simulink model "untitledtoch"  (R2016b)
settings: Solver=VariableStepAuto  StartTime=0  StopTime=20  MaxStep=0.001  RelTol=1e-3
libraries: simulink x1
settings Model: Creator=Admin  LastModifiedBy=Admin

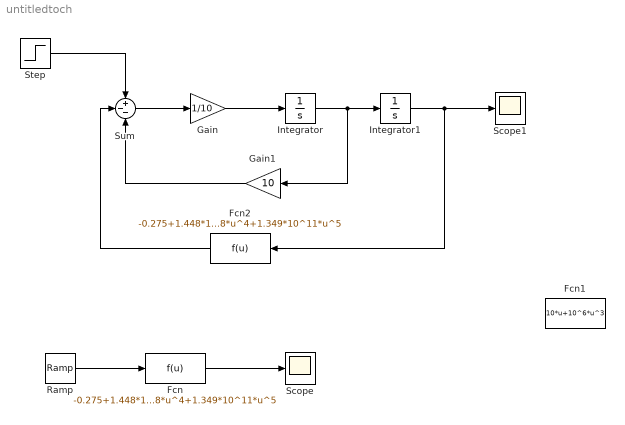
== system untitledtoch ==
  Fcn : Fcn  Expr=-0.275+1.448*10^3*u+-4.325*10^4*u^2+-1.543*10^7*u^3+2.141*10^8*u^4+1.349*10^11*u^5
  Fcn1 : Fcn  Expr=10*u+10^6*u^3
  Fcn2 : Fcn  Expr=-0.275+1.448*10^3*u+-4.325*10^4*u^2+-1.543*10^7*u^3+2.141*10^8*u^4+1.349*10^11*u^5
  Gain : Gain  Gain=1/10
  Gain1 : Gain  Gain=10
  Integrator : Integrator
  Integrator1 : Integrator
  Ramp : simulink/Sources/Ramp  slope=0.012  start=0  X0=-0.01
  Scope : Scope
  Scope1 : Scope
  Step : Step  Time=0  SampleTime=0
  Sum : Sum  Inputs=+--
  wires:
  Ramp/1 -> Fcn/1
  Fcn/1 -> Scope/1
  Step/1 -> Sum/1
  Sum/1 -> Gain/1
  Gain/1 -> Integrator/1
  Integrator/1 -> Gain1/1, Integrator1/1
  Integrator1/1 -> Fcn2/1, Scope1/1
  Gain1/1 -> Sum/3
  Fcn2/1 -> Sum/2
